simulink model "s_rotpen_bal"  (Simulink 10.3)
settings: Solver=ode1  StartTime=0.0  StopTime=10  FixedStep=0.001  RelTol=1e-3  EnableMultiTasking=on
values from neighbouring files (symbols this model uses):
  K = acker(A,B,DP)    [d_balance.m]    (also in setup_rotpen.m = d_balance(A, B, zeta, wn, p3, p4))
  wcf_1 = 2 * pi * 10.0    (= 62.8318530718)    [setup_rotpen.m]
  wcf_2 = 2 * pi * 10.0    (= 62.8318530718)    [setup_rotpen.m]
undefined symbols (not defined in the file or in its folder): A, B, C, D
libraries: simulink_extras x3
settings Model: Creator=MLevis  LastModifiedBy=WQ  ExtModeTrigDuration=10000
settings SolverCC: PositivePriorityOrder=on
settings OptimizationCC: BooleanDataType=off  OptimizeBlockIOStorage=off  BufferReuse=off  ExpressionFolding=off  LocalBlockOutputs=off  InitFltsAndDblsToZero=on
settings DebuggingCC: SaveWithParameterizedLinksMsg=none  SignalResolutionControl=TryResolveAllWithWarning  MultiTaskDSMMsg=warning  MultiTaskCondExecSysMsg=none
settings HardwareCC: TargetHWDeviceType=32-bit Generic
settings SFSimCC: SimUseLocalCustomCode=on  CustomCodeUndefinedFunction=FilterOut
settings RTWCC: Description=Quarc Win32 Target  SystemTargetFile=quarc_windows.tlc  TemplateMakefile=quarc_default_tmf  RTWUseLocalCustomCode=on
settings STFCustomTargetCC: TargetFcnLib=ansi_tfl_tmw.mat  TargetPreCompLibLocation=C:\DOCUME~1\ALLUSE~1\APPLIC~1\QUARC\lib\2007a\windows\release  CPPClassGenCompliant=on  SystemTargetFile=quarc_windows.tlc
settings GRTTargetCC: TargetFcnLib=ansi_tfl_tmw.mat  TargetPreCompLibLocation=C:\DOCUME~1\ALLUSE~1\APPLIC~1\QUARC\lib\2007a\windows\release  ParMdlRefBuildCompliant=off  CompOptLevelCompliant=off  ConcurrentExecutionCompliant=off  MatFileLogging=off  UseToolchainInfoCompliant=off  ExtMode=on  ExtModeMexFile=quarc_comm
settings ConfigComp: CovExternalEMLEnable=on

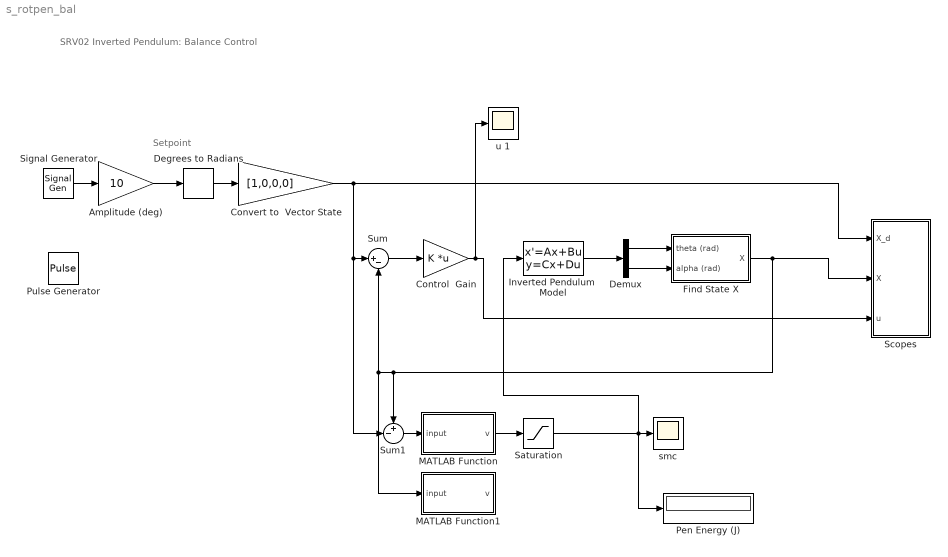
== system s_rotpen_bal ==
  note: Setpoint
  note: SRV02 Inverted Pendulum: Balance Control
  Amplitude (deg) : Gain  Gain=10  SaturateOnIntegerOverflow=on  OutDataTypeStr=Inherit: Same as input  ParamDataTypeStr=Inherit: Same as input
  Control  Gain : Gain  Gain=K  Multiplication=Matrix(K*u)
  Convert to  Vector State : Gain  Gain=[1,0,0,0]
  Degrees to Radians : simulink_extras/Transformations/Degrees to Radians
  Demux : Demux  Outputs=2
  Find State X : Subsystem
  Inverted Pendulum  Model : StateSpace  A=A  B=B  C=C  D=D  InitialCondition=[0 0.1 0 0]
  MATLAB Function : MATLAB Function  TreatAsAtomicUnit=on
  MATLAB Function1 : MATLAB Function  TreatAsAtomicUnit=on
  Pen Energy (J) : Display
      settings: Decimation=100
  Pulse Generator : DiscretePulseGenerator  PulseType=Time based  Period=10
  Saturation : Saturate  UpperLimit=10  LowerLimit=-10
  Scopes : Subsystem
  Signal Generator : SignalGenerator  WaveForm=square  Frequency=0.1
  Sum : Sum  Inputs=|+-
  Sum1 : Sum  Inputs=+-|
  "smc " : Scope
  u 1 : Scope
  wires:
  Amplitude (deg)/1 -> Degrees to Radians/1
  Degrees to Radians/1 -> Convert to  Vector State/1
  Convert to  Vector State/1 -> Scopes/1(X_d), Sum1/2, Sum/1
  Inverted Pendulum  Model/1 -> Demux/1
  Demux/1 -> Find State X/1(theta (rad))
  Demux/2 -> Find State X/2(alpha (rad))
  Sum/1 -> Control  Gain/1
  Control  Gain/1 -> u 1/1, Scopes/3(u)
  Find State X/1(X) -> Scopes/2(X), Sum1/1, MATLAB Function1/1(input), Sum/2
  Sum1/1 -> MATLAB Function/1(input)
  MATLAB Function/1(v) -> Saturation/1
  Signal Generator/1 -> Amplitude (deg)/1
  Saturation/1 -> Pen Energy (J)/1, "smc "/1, Inverted Pendulum  Model/1

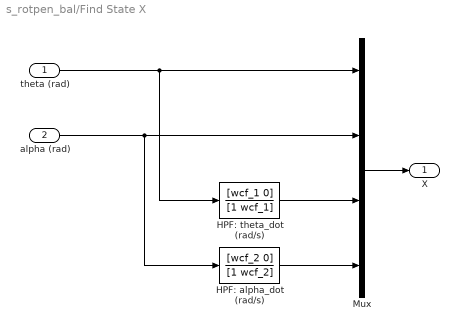
== system s_rotpen_bal/Find State X ==
  theta (rad) : Inport
  alpha (rad) : Inport  Port=2
  HPF: alpha_dot (rad/s) : TransferFcn  Numerator=[wcf_2 0]  Denominator=[1 wcf_2]
  HPF: theta_dot (rad/s) : TransferFcn  Numerator=[wcf_1 0]  Denominator=[1 wcf_1]
  Mux : Mux
  X : Outport
  wires:
  alpha (rad)/1 -> Mux/2, HPF: alpha_dot (rad/s)/1
  Mux/1 -> X/1
  theta (rad)/1 -> Mux/1, HPF: theta_dot (rad/s)/1
  HPF: theta_dot (rad/s)/1 -> Mux/3
  HPF: alpha_dot (rad/s)/1 -> Mux/4

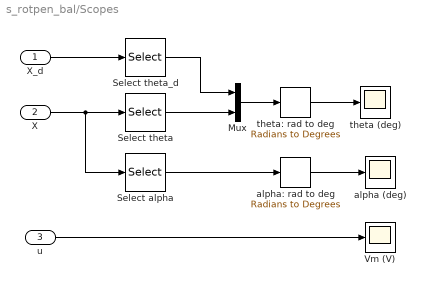
== system s_rotpen_bal/Scopes ==
  X_d : Inport
  X : Inport  Port=2
  u : Inport  Port=3
  Mux : Mux  Inputs=2
  Select alpha : Selector  InputPortWidth=4  IndexOptions=Index vector (dialog)  Indices=2  OutputSizes=[(-2)]
  Select theta : Selector  InputPortWidth=4  IndexOptions=Index vector (dialog)  Indices=1  OutputSizes=[(-2)]
  Select theta_d : Selector  InputPortWidth=4  IndexOptions=Index vector (dialog)  Indices=1  OutputSizes=[(-2)]
  Vm (V) : Scope
  alpha (deg) : Scope
  alpha: rad to deg : simulink_extras/Transformations/Radians to Degrees
  theta (deg) : Scope
  theta: rad to deg : simulink_extras/Transformations/Radians to Degrees
  wires:
  X_d/1 -> Select theta_d/1
  Select alpha/1 -> alpha: rad to deg/1
  X/1 -> Select alpha/1, Select theta/1
  Select theta_d/1 -> Mux/1
  u/1 -> Vm (V)/1
  alpha: rad to deg/1 -> alpha (deg)/1
  Mux/1 -> theta: rad to deg/1
  theta: rad to deg/1 -> theta (deg)/1
  Select theta/1 -> Mux/2

== matlab function MATLAB Function1 ==
  data: input input double; v output double
function v = fcn(input)
theta=input(1);
alpha=input(2);
dtheta=input(3);
dalpha=input(4);

%% Convert Angles to radians
% theta=theta*(pi/180);
% dtheta=dtheta*(pi/180);
% alpha=alpha*(pi/180);
% dalpha=dalpha*(pi/180);

%% Model Parameters
% kt=0.02797;
% km=0.02797;
% rm=3.3;
% L=0.153;
% r=0.08260;
% jeq=1.23*10^-4+0.00011;
% m=0.027;
% beq=0.0015;
Mp=0.1270;
Lr=0.2159;
Lp=0.3365;
Dp=0.0024;
Dr=0.0024;
Jp=0.0012;
g=9.8100;
eta_g=0.9000;
eta_m =0.6900;
Kg =70;
kt=0.0077;
Rm =2.6000;
km =0.0077;

%% Tuning Parameters
k=0.2;
lambda1=0.5;
lambda2=0.01;
lambda3=2;
phi=0.5;

%k=3;
%lambda1=0.5;
%lambda2=0.01;
%lambda3=10;
%phi=0.3;

%% Model

f2=81.4033*alpha-45.8259*dtheta-0.9319*dalpha;
g2=83.4659;
f1=122.0545*alpha-44.0966*dtheta-1.3972*dalpha;
g1=80.3162;

% a=jeq+m*r*r;
% b=m*L*r;
% c=4*m*L*L/3;
% d=m*9.81*L;
% g=(kt*km+beq*rm)/rm;
% f1=(-(b^2/2)*sin(2*alpha)*dalpha^2 - g*b*dtheta*cos(alpha) + a*d*sin(alpha))/(a*c-b^2*(cos(alpha))^2);
% g1=kt*b*cos(alpha)/(rm*(a*c-b^2*(cos(alpha))^2));
% f2=(c*f1-d*sin(alpha))/(b*cos(alpha));
% g2=kt*c/(rm*(a*c-b^2*(cos(alpha))^2));

%% Manifolds and Lyapunov Function
s1 = dalpha + lambda1*alpha;
s2 = dtheta + lambda3*theta;
v = abs(s1) + lambda2*abs(s2);

%% Saturation
if(phi<abs(v))
    out=v/phi;
else
    out=sign(v);
end

%% Output Voltage
v = (-k*out-(lambda1*dalpha+f1)*sign(s1)-lambda2*(lambda3*dtheta+f2)*sign(s2))/(g1*sign(s1)+lambda2*g2*sign(s2));

== matlab function MATLAB Function ==
  data: input input double; v output double
function v = fcn(input)
theta=input(1);
alpha=input(2);
dtheta=input(3);
dalpha=input(4);

%% Convert Angles to radians
% theta=theta*(pi/180);
% dtheta=dtheta*(pi/180);
% alpha=alpha*(pi/180);
% dalpha=dalpha*(pi/180);

%% Model Parameters
% kt=0.02797;
% km=0.02797;
% rm=3.3;
% L=0.153;
% r=0.08260;
% jeq=1.23*10^-4+0.00011;
% m=0.027;
% beq=0.0015;
Mp=0.1270;
Lr=0.2159;
Lp=0.3365;
Dp=0.0024;
Dr=0.0024;
Jp=0.0012;
g=9.8100;
eta_g=0.9000;
eta_m =0.6900;
Kg =70;
kt=0.0077;
Rm =2.6000;
km =0.0077;

%% Tuning Parameters

k=1.2;
lambda1=5.5;
lambda2=0.9;
lambda3=2.2;
phi=0.003;

% g
% k=1;
% lambda1=0.5;
% lambda2=0.01;
% lambda3=2;
% phi=0.5;

% k=1;
% lambda1=0.5;
% lambda2=0.01;
% lambda3=2;
% phi=0.5;

%k=3;
%lambda1=0.5;
%lambda2=0.01;
%lambda3=10;
%phi=0.3;

%% Model
a1=Mp*Lr^2+1/4*Mp*Lp^2-1/4*Mp*Lp^2*(cos(alpha))^2;
b1=-1/2*Mp*Lp*Lr*cos(alpha);
c1=-Dr*dtheta-0.5*Mp*Lp^2*sin(alpha)*cos(alpha)*dtheta*dalpha-0.5*Mp*Lp*Lr*sin(alpha)*dalpha^2;
a2=-0.5*Mp*Lp*Lr*cos(alpha);
b2=Jp+0.25*Mp*Lp^2;
c2=-Dp*dalpha+0.25*Mp*Lp^2*cos(alpha)*sin(alpha)*dtheta^2+0.5*Mp*Lp*g*sin(alpha);
c1=c1-eta_g*Kg*eta_m*kt*Kg*km*dtheta/Rm;

f2=(b2*c1-b1*c2)/(a1*b2-b1*a2);
g2=b2/(a1*b2-b1*a2);
f1=(-a2*c1+a1*c2)/(a1*b2-b1*a2);
g1=-a2/(a1*b2-b1*a2);
g2=g2*eta_g*Kg*eta_m*kt/Rm;
g1=g1*eta_g*Kg*eta_m*kt/Rm;

% a=jeq+m*r*r;
% b=m*L*r;
% c=4*m*L*L/3;
% d=m*9.81*L;
% g=(kt*km+beq*rm)/rm;
% f1=(-(b^2/2)*sin(2*alpha)*dalpha^2 - g*b*dtheta*cos(alpha) + a*d*sin(alpha))/(a*c-b^2*(cos(alpha))^2);
% g1=kt*b*cos(alpha)/(rm*(a*c-b^2*(cos(alpha))^2));
% f2=(c*f1-d*sin(alpha))/(b*cos(alpha));
% g2=kt*c/(rm*(a*c-b^2*(cos(alpha))^2));

%% Manifolds and Lyapunov Function
s1 = dalpha + lambda1*alpha;
s2 = dtheta + lambda3*theta;
v = abs(s1) + lambda2*abs(s2);

%% Saturation
if(phi<abs(v))
    out=v/phi;
else
    out=sign(v);
end

%% Output Voltage
v = (-k*out-(lambda1*dalpha+f1)*sign(s1)-lambda2*(lambda3*dtheta+f2)*sign(s2))/(g1*sign(s1)+lambda2*g2*sign(s2));
